simulink model "mech_interface_hyd_cylinder"  (Simulink 7.1)
settings: Solver=ode15s  StartTime=0.0  StopTime=10.0  RelTol=1e-3
model workspace (MAT data in the model file):
  a_a = 0.5
  a_b = 0.25
  a_c = 0.25
  b_a = 0.5
  b_b = 0.25
  b_c = 0.25
  Ma = 1
  Mb = 1
  Ia = [0.0416666666667  0  0; 0  0.104166666667  0; 0  0  0.104166666667]
  Ib = [0.0416666666667  0  0; 0  0.104166666667  0; 0  0  0.104166666667]
PostLoadFcn:
  | hws = get_param(gcs, 'modelworkspace');
  | 
  | hws.assignin('a_a', 0.5);
  | hws.assignin('a_b', 0.25);
  | hws.assignin('a_c', 0.25);
  | hws.assignin('b_a', 0.5);
  | hws.assignin('b_b', 0.25);
  | hws.assignin('b_c', 0.25);
  | 
  | hws.assignin('Ma', 1);
  | hws.assignin('Mb', 1);
  | 
  | hws.evalin('Ia = [1/3*Ma*(a_b^2 + a_c^2) 0 0;   0 1/3*Ma*(a_a^2 + a_c^2) 0;   0 0 1/3*Ma*(a_a^2 + a_b^2)];')
  | hws.evalin('Ib = [1/3*Mb*(b_b^2 + b_c^2) 0 0;   0 1/3*Mb*(b_a^2 + b_c^2) 0;   0 0 1/3*Mb*(b_a^2 + b_b^2)];')
  | 
  | clear hws
undefined symbols (not defined in the file or in its folder): sigbuilder_block
libraries: fl_lib x9, mblibv1 x8, nesl_utility x3
Description:
  | Hydraulic - 3D Translational Energy Conversion
  | 
  | The Translational Hydraulic Actuator subsystem uses a Prismatic -Translational Interface block and Translational Hydro-Mechanical Converter blocks to hydraulically actuate a prismatic joint.
  | 
  | The hydraulic part of the mechanism is modeled in Simscape. The rest of the mechanism is modeled in SimMechanics.
settings Model: Creator=ksanthan  LastModifiedBy=batserve  ExtModeAutoUpdateStatusClock=off
settings DataIOCC: SaveOutput=off  SignalLogging=off  SaveTime=off  OutputOption=SpecifiedOutputTimes  OutputTimes=[0:0.05:10]
settings DebuggingCC: AlgebraicLoopMsg=none  SolverPrmCheckMsg=none
settings GRTTargetCC: TargetFcnLib=ansi_tfl_tmw_new.mat
settings SimMechanicsCC: VisOnUpdateDiagram=on  VisDuringSimulation=on

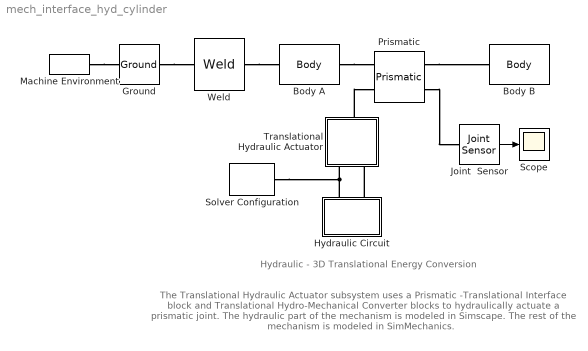
== system mech_interface_hyd_cylinder ==
  note: Hydraulic - 3D Translational Energy Conversion
  note: The Translational Hydraulic Actuator subsystem uses a Prismatic -Translational Interface block and
      | Translational Hydro-Mechanical Converter blocks to hydraulically actuate a prismatic joint.
      |
      | The hydraulic part of the mechanism is modeled in Simscape.
      | The rest of the mechanism is modeled in SimMechanics.
  Body A : mblibv1/Bodies/Body  DialogController=MECH.DynMechDlgSource  PhysicalDomain=mechanical  SubClassName=Unknown  LeftPortType=workingframe  RightPortType=workingframe  LConnTagsString=CS5  RConnTagsString=CS6  DialogClass=MechanicalBodyBlock  Mass=Ma  MassUnits=kg  InertiaUnits=kg*m^2  Inertia=Ia  Shape=Cylinder  ShapeDims=[1 1]  ShapeUnits=m  ShapeUse=false  Density=1  DensityUnits=kg/m^3  DensityUse=false  GraphicsMode=1  BodyColor=[0.5 0.5 0.5]  GraphicsObj=[]  AttachedToCS=1  CG=Left$CG$[a_a 0 0]$CS5$CS5$m$[0 0 0]$Euler X-Y-Z$deg$WORLD$false  WorkingFrames=Left$CS5$[0 0 0]$Adjoining$Adjoining$m$[0 0 0]$Euler X-Y-Z$deg$WORLD$true#Left$CS1$[0 -a_b 0]$CS5$CS5$m$[0 0 0]$Euler X-Y-Z$deg$WORLD$false#Right$CS2$[2*a_a -a_b 0]$CS5$CS5$m$[0 0 0]$Euler X-Y-Z$deg$WORLD$false#Right$CS6$[2*a_a 0 0]$CS5$CS5$m$[0 0 0]$Euler X-Y-Z$deg$WORLD$true#Right$CS3$[2*a_a a_b 0]$CS5$CS5$m$[0 0 0]$Euler X-Y-Z$deg$WORLD$false#Right$CS4$[0 a_b 0]$CS5$CS5$m$[0 0 0]$Euler X-Y-Z$deg$WORLD$false  CGPos=[a_a 0 0]  CGRot=[0 0 0]  CS0Pos=[]  CS0Rot=[]  CS1Pos=[0 -a_b 0]  CS1Rot=[0 0 0]  CS2Pos=[2*a_a -a_b 0]  CS2Rot=[0 0 0]  CS3Pos=[2*a_a a_b 0]  CS3Rot=[0 0 0]  CS4Pos=[0 a_b 0]  CS4Rot=[0 0 0]  CS5Pos=[0 0 0]  CS5Rot=[0 0 0]  CS6Pos=[2*a_a 0 0]  CS6Rot=[0 0 0]  CS7Pos=[]  CS7Rot=[]  CS8Pos=[]  CS8Rot=[]  CS9Pos=[]  CS9Rot=[]  CS10Pos=[]  CS10Rot=[]  CS11Pos=[]  CS11Rot=[]  CS12Pos=[]  CS12Rot=[]  CS13Pos=[]  CS13Rot=[]  CS14Pos=[]  CS14Rot=[]  CS15Pos=[]  CS15Rot=[]  CS16Pos=[]  CS16Rot=[]  CS17Pos=[]  CS17Rot=[]  CS18Pos=[]  CS18Rot=[]  CS19Pos=[]  CS19Rot=[]  CS20Pos=[]  CS20Rot=[]
  Body B : mblibv1/Bodies/Body  DialogController=MECH.DynMechDlgSource  PhysicalDomain=mechanical  SubClassName=Unknown  LeftPortType=workingframe  RightPortType=workingframe  LConnTagsString=CS5  DialogClass=MechanicalBodyBlock  Mass=Mb  MassUnits=kg  InertiaUnits=kg*m^2  Inertia=Ib  Shape=Cylinder  ShapeDims=[1 1]  ShapeUnits=m  ShapeUse=false  Density=1  DensityUnits=kg/m^3  DensityUse=false  GraphicsMode=1  BodyColor=[0.5 0.5 0.5]  GraphicsObj=[]  AttachedToCS=1  CG=Left$CG$[b_a 0 0]$CS5$CS5$m$[0 0 0]$Euler X-Y-Z$deg$WORLD$false  WorkingFrames=Left$CS5$[b_a 0 0]$Adjoining$Adjoining$m$[0 0 0]$Euler X-Y-Z$deg$WORLD$true#Left$CS1$[0 -b_b 0]$CS5$CS5$m$[0 0 0]$Euler X-Y-Z$deg$WORLD$false#Right$CS2$[2*b_a -b_b 0]$CS5$CS5$m$[0 0 0]$Euler X-Y-Z$deg$WORLD$false#Right$CS6$[2*b_a 0 0]$CS5$CS5$m$[0 0 0]$Euler X-Y-Z$deg$WORLD$false#Right$CS3$[2*b_a b_b 0]$CS5$CS5$m$[0 0 0]$Euler X-Y-Z$deg$WORLD$false#Right$CS4$[0 b_b 0]$CS5$CS5$m$[0 0 0]$Euler X-Y-Z$deg$WORLD$false  CGPos=[b_a 0 0]  CGRot=[0 0 0]  CS0Pos=[]  CS0Rot=[]  CS1Pos=[0 -b_b 0]  CS1Rot=[0 0 0]  CS2Pos=[2*b_a -b_b 0]  CS2Rot=[0 0 0]  CS3Pos=[2*b_a b_b 0]  CS3Rot=[0 0 0]  CS4Pos=[0 b_b 0]  CS4Rot=[0 0 0]  CS5Pos=[b_a 0 0]  CS5Rot=[0 0 0]  CS6Pos=[2*b_a 0 0]  CS6Rot=[0 0 0]  CS7Pos=[]  CS7Rot=[]  CS8Pos=[]  CS8Rot=[]  CS9Pos=[]  CS9Rot=[]  CS10Pos=[]  CS10Rot=[]  CS11Pos=[]  CS11Rot=[]  CS12Pos=[]  CS12Rot=[]  CS13Pos=[]  CS13Rot=[]  CS14Pos=[]  CS14Rot=[]  CS15Pos=[]  CS15Rot=[]  CS16Pos=[]  CS16Rot=[]  CS17Pos=[]  CS17Rot=[]  CS18Pos=[]  CS18Rot=[]  CS19Pos=[]  CS19Rot=[]  CS20Pos=[]  CS20Rot=[]
  Ground : mblibv1/Bodies/Ground  DialogController=MECH.DynMechDlgSource  SystemSampleTime=-1  LeftPortType=env  RightPortType=workingframe  PhysicalDomain=Mechanical  DialogClass=GroundBlock  CoordPosition=[0 0 0]  CoordPositionUnits=m  StateVectorMgrId=-1  MachineId=[0 0]  ShowEnvPort=on
  Hydraulic Circuit : Subsystem  Orientation=up
  Joint  Sensor : mblibv1/Sensors &  Actuators/Joint Sensor  DialogController=MECH.DynMechDlgSource  SystemSampleTime=-1  PhysicalDomain=Mechanical  PortType=blob  Muxed=on  Pose=off  Angle=on  AngleUnits=deg  ArcVelocity=off  ArcVelocityUnits=deg/s  ArcAcceleration=off  ArcAccelerationUnits=deg/s^2  CoordPosition=on  CoordPositionUnits=m  Velocity=off  VelocityUnits=m/s  Acceleration=off  AccelerationUnits=m/s^2  Quaternion=on  QuaternionDT=off  QuaternionDDT=off  QuaternionUnits=off  OutputVector=[1]  ActiveIO=on  Width=1  DialogClass=MechanicalSensorBlock  Primitive=P1  Force=off  ForceUnits=N  Torque=off  TorqueUnits=N*m  ReferenceFrame=Absolute (World)  ReactionSensedSide=Base  ReactionReferenceFrame=Absolute (World)  ReactionForce=off  ReactionForceUnits=N  ReactionMoment=off  ReactionMomentUnits=N*m
  Machine Environment : mblibv1/Bodies/Machine Environment  Tag=Factory ground  DialogController=MECH.DialogSource  SystemSampleTime=-1  PortType=env  PhysicalDomain=Mechanical  DialogTemplateClass=MECH.MachineEnvironment  SyncWhenCopied=off  Gravity=[0 -9.81 0]  GravityUnits=m/s^2  GravityAsSignal=off  Dimensionality=Auto-detect  AnalysisType=Forward dynamics  LinearAssemblyTolerance=1e-3  LinearAssemblyToleranceUnits=m  AngularAssemblyTolerance=1e-3  AngularAssemblyToleranceUnits=rad  ConstraintSolverType=Stabilizing  ConstraintRelTolerance=1e-4  ConstraintAbsTolerance=1e-4  UseRobustSingularityHandling=off  RedundancyAnalysisToleranceType=Automatically select tolerance  RedundancyAnalysisTolerance=1e-14  StatePerturbationType=Fixed  PerturbationSize=1e-5  VisualizeMachine=on
  Prismatic : mblibv1/Joints/Prismatic  DialogController=MECH.DynMechDlgSource  PhysicalDomain=mechanical  SubClassName=Unknown  LeftPortType=blob  RightPortType=blob  LConnTagsString=__newl0|SA1  RConnTagsString=__newr0|SA1  NumSAPorts=2  CutJoint=off  MarkAsCut=off  Primitives=prismatic  PrimitiveProps=P1$World$[1 0 0]$prismatic  DialogClass=JointBlock  P1Axis=[1 0 0]
  Scope : Scope
      settings: TimeRange=10  YMin=-0.2  YMax=1.4
  Solver Configuration : nesl_utility/Solver Configuration  DialogController=NetworkEngine.DynNeUtilDlgSource  SystemSampleTime=-1  PhysicalDomain=network_engine_domain  LeftPortType=input  RightPortType=generic  SubClassName=solver  Accelerate=off  Profile=off  ResidualTolerance=1e-9  MaxNonlinIter=12  MaxModeIter=2  DoFixedCost=off  DoDC=off  LinearAlgebra=Sparse
  Translational Hydraulic Actuator : Subsystem  Orientation=up
  Weld : mblibv1/Joints/Weld  DialogController=MECH.DynMechDlgSource  PhysicalDomain=mechanical  SubClassName=Unknown  LeftPortType=blob  RightPortType=blob  LConnTagsString=__newl0  RConnTagsString=__newr0  NumSAPorts=0  CutJoint=off  MarkAsCut=off  Primitives=weld  PrimitiveProps=W$World$[0 0 0]$weld  DialogClass=JointBlock  WAxis=[0 0 0]
  wires:
  Joint  Sensor/1 -> Scope/1
  connections:
  Ground/RConn1 -- Weld/LConn1
  Prismatic/RConn1 -- Body B/LConn1
  Weld/RConn1 -- Body A/LConn1
  Machine Environment/RConn1 -- Ground/LConn1
  Prismatic/RConn2 -- Joint  Sensor/LConn1
  Translational Hydraulic Actuator/LConn1 -- Hydraulic Circuit/RConn1 -- Solver Configuration/RConn1
  Hydraulic Circuit/RConn2 -- Translational Hydraulic Actuator/LConn2
  Body A/RConn1 -- Prismatic/LConn1
  Translational Hydraulic Actuator/RConn1 -- Prismatic/LConn2

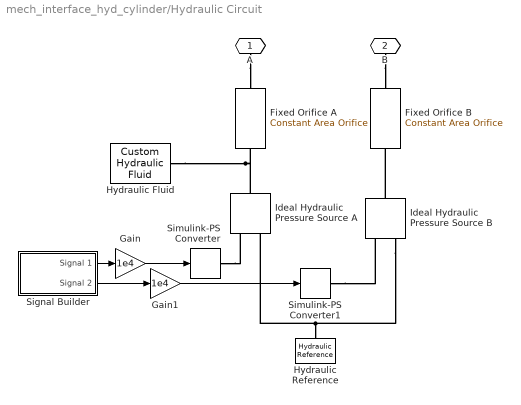
== system mech_interface_hyd_cylinder/Hydraulic Circuit ==
  Fixed Orifice A : fl_lib/Hydraulic/Hydraulic Elements/Constant Area Orifice  Orientation=up  DialogController=NetworkEngine.DynNeDlgSource  SystemSampleTime=-1  area=1e-04 m^2  C_d=0.7  Re_cr=12  flow_rate_Log=off  pr_drop_Log=off  power_Log=off  LocalVarNames=|flow_rate|pr_drop|Re|power  LocalVarDescs=|Flow rate through the orifice (m^3/s)|Pressure drop across the orifice (Pa)|Reynolds number|Power (W)  LocalVarLogging=[0 0 0 0]
  Fixed Orifice B : fl_lib/Hydraulic/Hydraulic Elements/Constant Area Orifice  Orientation=down  DialogController=NetworkEngine.DynNeDlgSource  SystemSampleTime=-1  area=1e-04 m^2  C_d=0.7  Re_cr=12  flow_rate_Log=off  pr_drop_Log=off  power_Log=off  LocalVarNames=|flow_rate|pr_drop|Re|power  LocalVarDescs=|Flow rate through the orifice (m^3/s)|Pressure drop across the orifice (Pa)|Reynolds number|Power (W)  LocalVarLogging=[0 0 0 0]
  Gain : Gain  Gain=1e4  ParameterDataType=sfix(16)  ParameterScaling=2^0  OutDataType=sfix(16)  OutScaling=2^0
  Gain1 : Gain  Gain=1e4  ParameterDataType=sfix(16)  ParameterScaling=2^0  OutDataType=sfix(16)  OutScaling=2^0
  Hydraulic Fluid : fl_lib/Hydraulic/Hydraulic Utilities/Custom Hydraulic Fluid  DialogController=NetworkEngine.DynNeDlgSource  SystemSampleTime=-1  density=961.873 kg/m^3  viscosity_kin=7.12831 cSt  bulk=1.24285e+09 Pa  alpha=0.005  LocalVarLogging=[]
  Hydraulic Reference : fl_lib/Hydraulic/Hydraulic Elements/Hydraulic Reference  Orientation=down  DialogController=NetworkEngine.DynNeDlgSource  SystemSampleTime=-1  LocalVarLogging=[]
  Ideal Hydraulic Pressure Source A : fl_lib/Hydraulic/Hydraulic Sensors and Sources/Ideal Hydraulic Pressure Source  Orientation=down  DialogController=NetworkEngine.DynNeDlgSource  SystemSampleTime=-1  flow_rate_Log=off  pr_differential_Log=off  power_Log=off  LocalVarNames=|flow_rate|pr_differential|power  LocalVarDescs=|Flow rate through the source (m^3/s)|Pressure differential across the source (Pa)|Source power (W)  LocalVarLogging=[0 0 0]
  Ideal Hydraulic Pressure Source B : fl_lib/Hydraulic/Hydraulic Sensors and Sources/Ideal Hydraulic Pressure Source  Orientation=down  DialogController=NetworkEngine.DynNeDlgSource  SystemSampleTime=-1  flow_rate_Log=off  pr_differential_Log=off  power_Log=off  LocalVarNames=|flow_rate|pr_differential|power  LocalVarDescs=|Flow rate through the source (m^3/s)|Pressure differential across the source (Pa)|Source power (W)  LocalVarLogging=[0 0 0]
  Signal Builder : Subsystem  Tag=STV Subsys  LoadFcn=sigbuilder_block('load');  StartFcn=sigbuilder_block('start');  StopFcn=sigbuilder_block('stop');  ClipboardFcn=sigbuilder_block('clipboard');  mask(Sigbuilder block){}
      mask help: Sigbuilder GUI
      mask init:
      | if ~strcmp(get_param(bdroot(gcbh),'SimulationStatus'),'stopped') tuvar = sigbuilder_block('maskInit'); end
      settings: CopyFcn=sigbuilder_block('copy');  DeleteFcn=sigbuilder_block('delete');  ModelCloseFcn=sigbuilder_block('modelClose');  PreSaveFcn=sigbuilder_block('preSave');  NameChangeFcn=sigbuilder_block('namechange');  OpenFcn=sigbuilder_block('open',[46.5 475.5 550.5 371.25 ]);  CloseFcn=sigbuilder_block('close');
      mask Display: plot(0,0,100,100,[10,10,40,40,10],[80,20,20,80,80],[40,10],[50,50], [40,27,10],[65,72,56],[40,25,25,10],[28,28,43,43]);
  Simulink-PS Converter : nesl_utility/Simulink-PS Converter  DialogController=NetworkEngine.DynNeUtilDlgSource  SystemSampleTime=-1  PhysicalDomain=network_engine_domain  LeftPortType=input  RightPortType=output  SubClassName=ps_input  Unit=N/m^2  AffineConversion=off
  Simulink-PS Converter1 : nesl_utility/Simulink-PS Converter  DialogController=NetworkEngine.DynNeUtilDlgSource  SystemSampleTime=-1  PhysicalDomain=network_engine_domain  LeftPortType=input  RightPortType=output  SubClassName=ps_input  Unit=N/m^2  AffineConversion=off
  A : PMIOPort  Orientation=down  Port=1  Side=Right
  B : PMIOPort  Orientation=down  Port=2  Side=Right
  wires:
  Signal Builder/2(Signal 2) -> Gain1/1
  Signal Builder/1(Signal 1) -> Gain/1
  Gain/1 -> Simulink-PS Converter/1
  Gain1/1 -> Simulink-PS Converter1/1
  connections:
  Ideal Hydraulic Pressure Source B/LConn1 -- Fixed Orifice B/RConn1
  Hydraulic Fluid/RConn1 -- Ideal Hydraulic Pressure Source A/LConn1 -- Fixed Orifice A/LConn1
  Simulink-PS Converter/RConn1 -- Ideal Hydraulic Pressure Source A/RConn1
  Simulink-PS Converter1/RConn1 -- Ideal Hydraulic Pressure Source B/RConn1
  A/RConn1 -- Fixed Orifice A/RConn1
  B/RConn1 -- Fixed Orifice B/LConn1
  Ideal Hydraulic Pressure Source B/RConn2 -- Ideal Hydraulic Pressure Source A/RConn2 -- Hydraulic Reference/LConn1

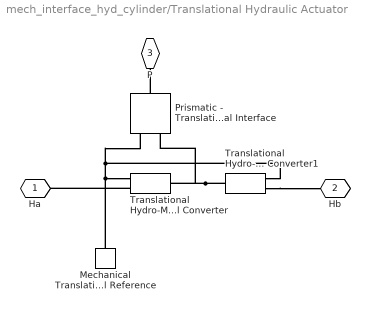
== system mech_interface_hyd_cylinder/Translational Hydraulic Actuator ==
  Mechanical Translational Reference : fl_lib/Mechanical/Translational Elements/Mechanical Translational Reference  Orientation=down  DialogController=NetworkEngine.DynNeDlgSource  SystemSampleTime=-1  LocalVarLogging=[]
  Prismatic - Translational Interface : mblibv1/Interface  Elements/Prismatic - Translational Interface  Orientation=up  DialogController=MECH.DynMechDlgSource  SystemSampleTime=-1  DialogClass=PrismaticTranslationalInterface  Primitive=P1
  Translational Hydro-Mechanical Converter : fl_lib/Hydraulic/Hydraulic Elements/Translational Hydro-Mechanical Converter  DialogController=NetworkEngine.DynNeDlgSource  SystemSampleTime=-1  area=5e-04 m^2  or=1  flow_rate_Log=off  pressure_Log=off  force_Log=off  power_Log=off  LocalVarNames=|flow_rate|pressure|force|power  LocalVarDescs=|Flow rate into the chamber (m^3/s)|Pressure at the inlet (Pa)|Output force (N)|Power (W)  LocalVarLogging=[0 0 0 0]
  Translational Hydro-Mechanical Converter1 : fl_lib/Hydraulic/Hydraulic Elements/Translational Hydro-Mechanical Converter  Orientation=left  DialogController=NetworkEngine.DynNeDlgSource  SystemSampleTime=-1  area=5e-04 m^2  or=2  flow_rate_Log=off  pressure_Log=off  force_Log=off  power_Log=off  LocalVarNames=|flow_rate|pressure|force|power  LocalVarDescs=|Flow rate into the chamber (m^3/s)|Pressure at the inlet (Pa)|Output force (N)|Power (W)  LocalVarLogging=[0 0 0 0]
  Ha : PMIOPort  Tag=PMCPort  Port=1  Side=Left
  Hb : PMIOPort  Tag=PMCPort  Orientation=left  Port=2  Side=Left
  P : PMIOPort  Tag=PMCPort  Orientation=down  Port=3  Side=Right
  connections:
  Prismatic - Translational Interface/LConn1 -- Mechanical Translational Reference/LConn1 -- Translational Hydro-Mechanical Converter/LConn1 -- Translational Hydro-Mechanical Converter1/LConn1
  Translational Hydro-Mechanical Converter/LConn2 -- Ha/RConn1
  Translational Hydro-Mechanical Converter1/LConn2 -- Hb/RConn1
  Prismatic - Translational Interface/RConn1 -- P/RConn1
  Prismatic - Translational Interface/LConn2 -- Translational Hydro-Mechanical Converter1/RConn1 -- Translational Hydro-Mechanical Converter/RConn1

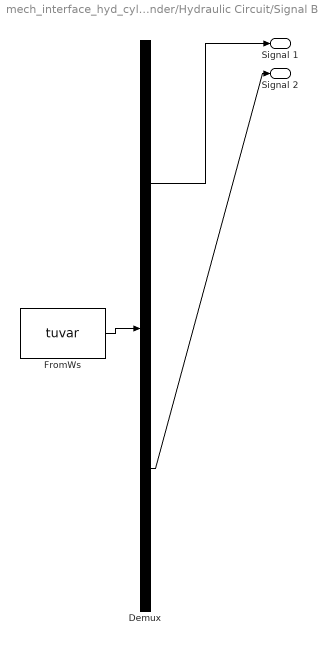
== system mech_interface_hyd_cylinder/Hydraulic Circuit/Signal Builder ==
  Demux : Demux  Tag=STV Demux  Outputs=2
  FromWs : FromWorkspace  Tag=STV FromWs  VariableName=tuvar  SampleTime=0  SigBuilderData=DataTag2  VnvData=DataTag3
      SigBuilderData=|
      | channels(1).label = 'Signal 1'
      | channels(1).allXData = {[0 1.02 1.02 2 3 4 5.02 10]}
      | channels(1).allYData = {[0 0 0.01 1 1 1 0.01 0]}
      | channels(2).label = 'Signal 2'
      | channels(2).allXData = {[0 4 5 6.98 7.98 10]}
      | channels(2).allYData = {[0 0 0.99 0.99396 0 0]}
      | common.afterFinalStr = 'Extrapolate'
      | common.sampleTime = 0
      | dataSet.timeRange = [0 10]
      | dataSet.name = 'Group 1'
  Signal 1 : Outport  Tag=STV Outport  OutDataType=sfix(16)  OutScaling=2^0
  Signal 2 : Outport  Tag=STV Outport  Port=2  OutDataType=sfix(16)  OutScaling=2^0
  wires:
  Demux/1 -> Signal 1/1
  FromWs/1 -> Demux/1
  Demux/2 -> Signal 2/1
